simulink model "model"  (R2021a)
settings: Solver=VariableStepAuto  StartTime=0.0  StopTime=100  FixedStep=0.001  RelTol=1e-3
settings Model: Creator=benal  LastModifiedBy=benal

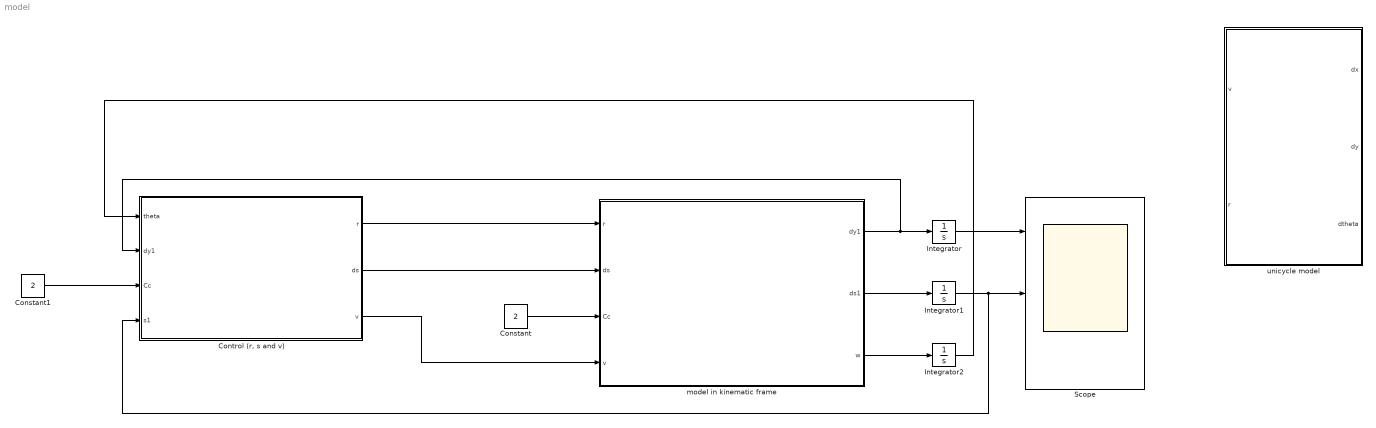
== system model ==
  Constant : Constant  Value=2
  Constant1 : Constant  Value=2
  "Control (r, s and v)" : Subsystem
  Integrator : Integrator  InitialCondition=1
  Integrator1 : Integrator  InitialCondition=2
  Integrator2 : Integrator  InitialCondition=pi/6
  Scope : Scope  NumInputPorts=3
  model in kinematic frame : Subsystem
  unicycle model : Subsystem
  wires:
  "Control (r, s and v)"/1(r) -> model in kinematic frame/1(r)
  "Control (r, s and v)"/2(ds) -> model in kinematic frame/2(ds)
  "Control (r, s and v)"/3(v) -> model in kinematic frame/4(v)
  Constant/1 -> model in kinematic frame/3(Cc)
  model in kinematic frame/1(dy1) -> "Control (r, s and v)"/2(dy1), Integrator/1
  model in kinematic frame/2(ds1) -> Integrator1/1
  model in kinematic frame/3(w) -> Integrator2/1
  Integrator1/1 -> "Control (r, s and v)"/4(s1), Scope/2
  Integrator/1 -> Scope/1
  Integrator2/1 -> "Control (r, s and v)"/1(theta)
  Constant1/1 -> "Control (r, s and v)"/3(Cc)

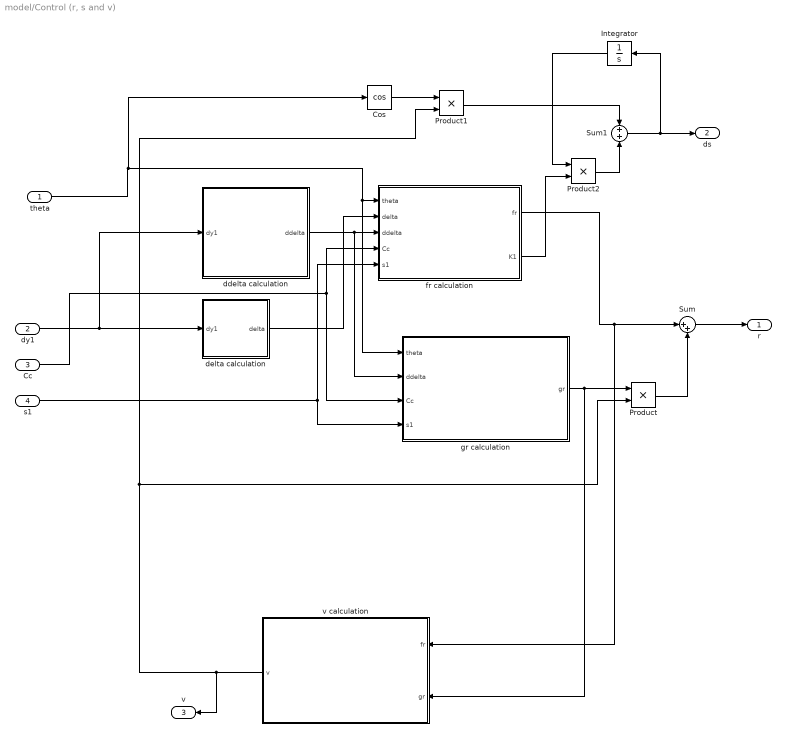
== system model/Control (r, s and v) ==
  theta : Inport
  dy1 : Inport  Port=2
  Cc : Inport  Port=3
  s1 : Inport  Port=4
  Cos : Trigonometry  Operator=cos
  Integrator : Integrator
  Product : Product
  Product1 : Product
  Product2 : Product
  Sum : Sum  Inputs=|++
  Sum1 : Sum
  ddelta calculation : Subsystem
  delta calculation : Subsystem
  fr calculation : MATLAB Function  TreatAsAtomicUnit=on
  gr calculation : MATLAB Function  TreatAsAtomicUnit=on
  v calculation : MATLAB Function  TreatAsAtomicUnit=on
  r : Outport
  ds : Outport  Port=2
  v : Outport  Port=3
  wires:
  Cc/1 -> fr calculation/4(Cc), gr calculation/3(Cc)
  v calculation/1(v) -> v/1, Product1/2, Product/2
  s1/1 -> gr calculation/4(s1), fr calculation/5(s1)
  dy1/1 -> ddelta calculation/1(dy1), delta calculation/1(dy1)
  ddelta calculation/1(ddelta) -> gr calculation/2(ddelta), fr calculation/3(ddelta)
  Product/1 -> Sum/2
  theta/1 -> Cos/1, gr calculation/1(theta), fr calculation/1(theta)
  Sum/1 -> r/1
  delta calculation/1(delta) -> fr calculation/2(delta)
  fr calculation/1(fr) -> v calculation/1(fr), Sum/1
  gr calculation/1(gr) -> v calculation/2(gr), Product/1
  Cos/1 -> Product1/1
  Product1/1 -> Sum1/1
  Product2/1 -> Sum1/2
  fr calculation/2(K1) -> Product2/2
  Sum1/1 -> Integrator/1, ds/1
  Integrator/1 -> Product2/1

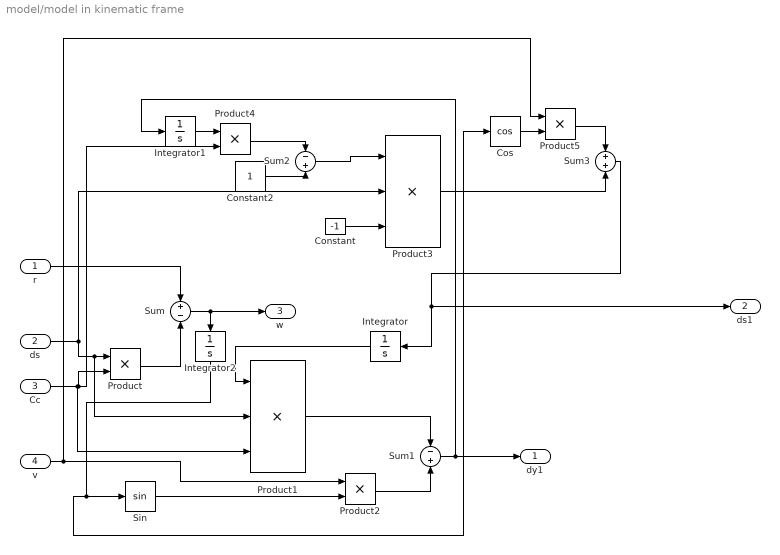
== system model/model in kinematic frame ==
  r : Inport
  ds : Inport  Port=2
  Cc : Inport  Port=3
  v : Inport  Port=4
  Constant : Constant  Value=-1
  Constant2 : Constant
  Cos : Trigonometry  Operator=cos
  Integrator : Integrator  InitialCondition=1
  Integrator1 : Integrator  InitialCondition=2
  Integrator2 : Integrator  InitialCondition=pi/6
  Product{,2,4..5} (4 alike) : Product
  Product1 : Product  Inputs=3
  Product3 : Product  Inputs=3
  Sin : Trigonometry
  Sum : Sum  Inputs=+-
  Sum1 : Sum  Inputs=-+
  Sum2 : Sum  Inputs=-+
  Sum3 : Sum
  dy1 : Outport
  ds1 : Outport  Port=2
  w : Outport  Port=3
  wires:
  Product/1 -> Sum/2
  v/1 -> Product2/1, Product5/1
  r/1 -> Sum/1
  Cc/1 -> Product4/2, Product/2, Product1/3
  Constant2/1 -> Sum2/2
  Integrator/1 -> Product1/1
  Cos/1 -> Product5/2
  Product5/1 -> Sum3/1
  Product3/1 -> Sum3/2
  Sum3/1 -> ds1/1, Integrator/1
  ds/1 -> Product3/2, Product1/2, Product/1
  Sum1/1 -> dy1/1, Integrator1/1
  Product1/1 -> Sum1/1
  Product4/1 -> Sum2/1
  Integrator2/1 -> Cos/1, Sin/1
  Sum/1 -> w/1, Integrator2/1
  Constant/1 -> Product3/3
  Product2/1 -> Sum1/2
  Sum2/1 -> Product3/1
  Sin/1 -> Product2/2
  Integrator1/1 -> Product4/1

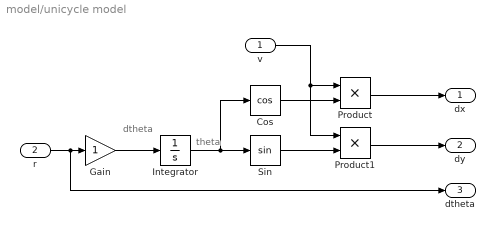
== system model/unicycle model ==
  note: theta
  note: dtheta
  v : Inport
  r : Inport  Port=2
  Cos : Trigonometry  Operator=cos
  Gain : Gain
  Integrator : Integrator
  Product : Product
  Product1 : Product
  Sin : Trigonometry
  dx : Outport
  dy : Outport  Port=2
  dtheta : Outport  Port=3
  wires:
  Integrator/1 -> Sin/1, Cos/1
  Product1/1 -> dy/1
  r/1 -> dtheta/1, Gain/1
  v/1 -> Product1/1, Product/1
  Sin/1 -> Product1/2
  Gain/1 -> Integrator/1
  Cos/1 -> Product/2
  Product/1 -> dx/1

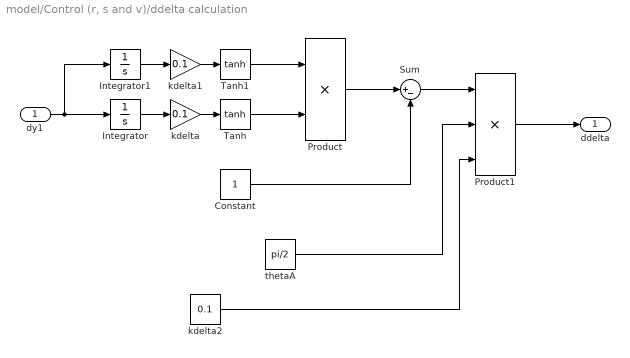
== system model/Control (r, s and v)/ddelta calculation ==
  dy1 : Inport
  Constant : Constant
  Integrator : Integrator
  Integrator1 : Integrator
  Product : Product
  Product1 : Product  Inputs=3
  Sum : Sum  Inputs=|+-
  Tanh : Trigonometry  Operator=tanh
  Tanh1 : Trigonometry  Operator=tanh
  kdelta : Gain  Gain=0.1
  kdelta1 : Gain  Gain=0.1
  kdelta2 : Constant  Value=0.1
  thetaA : Constant  Value=pi/2
  ddelta : Outport
  wires:
  thetaA/1 -> Product1/2
  Tanh/1 -> Product/2
  kdelta1/1 -> Tanh1/1
  kdelta/1 -> Tanh/1
  kdelta2/1 -> Product1/3
  Integrator/1 -> kdelta/1
  dy1/1 -> Integrator1/1, Integrator/1
  Integrator1/1 -> kdelta1/1
  Product/1 -> Sum/1
  Tanh1/1 -> Product/1
  Product1/1 -> ddelta/1
  Constant/1 -> Sum/2
  Sum/1 -> Product1/1

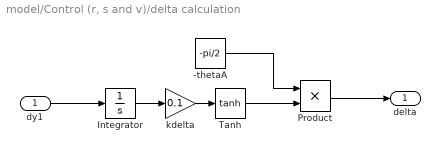
== system model/Control (r, s and v)/delta calculation ==
  dy1 : Inport
  -thetaA : Constant  Value=-pi/2
  Integrator : Integrator
  Product : Product
  Tanh : Trigonometry  Operator=tanh
  kdelta : Gain  Gain=0.1
  delta : Outport
  wires:
  Integrator/1 -> kdelta/1
  Tanh/1 -> Product/2
  Product/1 -> delta/1
  dy1/1 -> Integrator/1
  -thetaA/1 -> Product/1
  kdelta/1 -> Tanh/1

== matlab function model/Control (r, s and v)/gr calculation ==
  data: theta input; gr output; ddelta input; Cc input; s1 input
function gr = fcn(theta,ddelta,Cc,s1)

gr = Cc*cos(theta)*(1-s1*ddelta)+ddelta*sin(theta);

== matlab function model/Control (r, s and v)/fr calculation ==
  data: theta input; fr output; delta input; ddelta input; Cc input; s1 input; K1 output
function [fr,K1] = fcn(theta,delta,ddelta,Cc,s1)
k1 = 1;
k2 = 1;

K1 = k1/(1+(s1*Cc*(1-s1*ddelta))^2);

fr = -k2*tanh(theta-delta)+K1*s1*Cc*(1-s1*ddelta);

== matlab function model/Control (r, s and v)/v calculation ==
  data: fr input; v output; gr input
function v = fcn(fr,gr)
wmax = 2*pi;
R = 0.1;
L = 0.15;
vmax = 6;
v = (R*wmax-L*(1/4+fr^2))/(1+L*(1/4+gr^2));
v = min(v,vmax);
